simulink model "LQR_Control_Model"  (R2018b)
settings: Solver=ode1  StartTime=0.0  StopTime=15  FixedStep=0.001  MaxStep=0.001  RelTol=1e-3
values from neighbouring files (symbols this model uses):
  K = 0.2    [SingleNN_Delta.m]    (also in SingleNN_Hebb.m)
undefined symbols (not defined in the file or in its folder): sigbuilder_block
settings Model: Creator=Lenovo  LastModifiedBy=Richard
settings DataIOCC: LimitDataPoints=on  SaveFormat=Array
settings OptimizationCC: BlockReduction=off  BooleanDataType=off  LifeSpan=inf
settings DebuggingCC: SaveWithParameterizedLinksMsg=none  UnderspecifiedInitializationDetection=Classic  MergeDetectMultiDrivingBlocksExec=none  SignalResolutionControl=TryResolveAllWithWarning  SFUnexpectedBacktrackingDiag=warning  SFNoUnconditionalDefaultTransitionDiag=warning  SFExecutionAtInitializationDiag=none
settings HardwareCC: ProdBitPerPointer=32  ProdBitPerSizeT=32  ProdBitPerPtrDiffT=32  ProdLargestAtomicFloat=None  ProdIntDivRoundTo=Undefined  ProdEndianess=Unspecified  ProdWordSize=32  ProdHWDeviceType=32-bit Generic  TargetUnknown=on
settings ModelReferenceCC: PropagateSignalLabelsOutOfModel=off
settings SFSimCC: SimUseLocalCustomCode=off
settings RTWCC: RTWUseLocalCustomCode=off
settings CodeAppCC: StateflowObjectComments=on
settings GRTTargetCC: TargetLangStandard=C89/C90 (ANSI)  GeneratePreprocessorConditionals=Disable all
settings ConfigComp: CovMetricSettings=dw  CovHtmlReporting=on  CovSaveCumulativeToWorkspaceVar=on  CovSaveSingleToWorkspaceVar=on  CovExternalEMLEnable=off  CovSFcnEnable=off

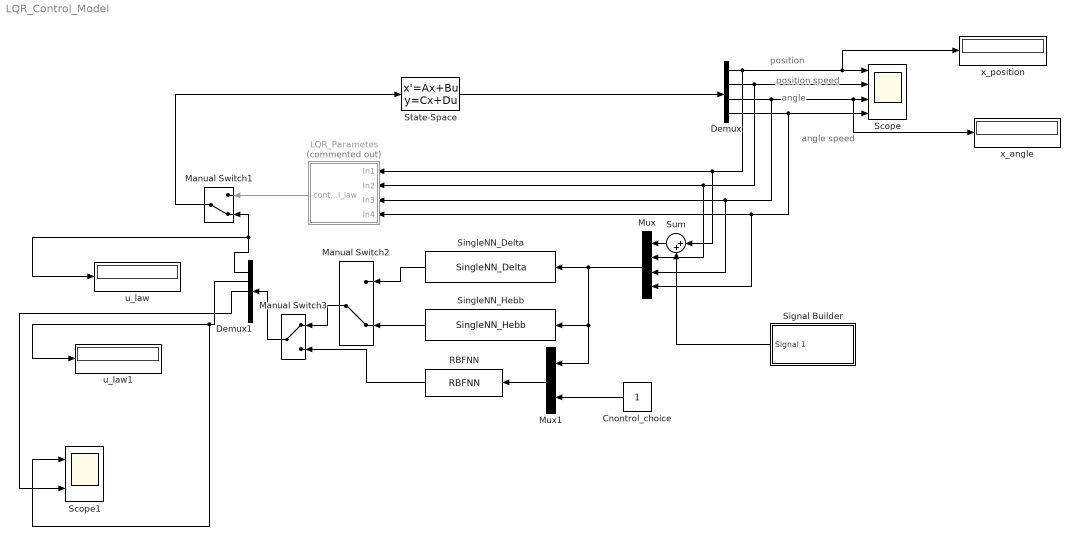
== system LQR_Control_Model ==
  note: angle speed
  note: angle
  note: position speed
  note: position
  Cnontrol_choice : Constant
  Demux : Demux
  Demux1 : Demux  Outputs=5
  LQR_Parametes : Subsystem  Commented=on
  Manual Switch1 : ManualSwitch  CurrentSetting=0
  Manual Switch2 : ManualSwitch  CurrentSetting=0
  Manual Switch3 : ManualSwitch
  Mux : Mux
  Mux1 : Mux  Inputs=2
  RBFNN : S-Function  FunctionName=RBFNN  SFunctionDeploymentMode=off  EnableBusSupport=off
  Scope : Scope  NumInputPorts=4
  Scope1 : Scope  NumInputPorts=2
  Signal Builder : Subsystem  Tag=STV Subsys  LoadFcn=sigbuilder_block('load',[437.6 199.2 550.4 400 ]);  StartFcn=sigbuilder_block('start');  StopFcn=sigbuilder_block('stop');  ClipboardFcn=sigbuilder_block('clipboard');  mask(Sigbuilder block){tuvar=[0:10]}
      mask help: Simulink:masks:SigbuilderBlock_MD
      mask init:
      | if ~strcmp(get_param(bdroot(gcbh),'SimulationStatus'),'stopped') tuvar = sigbuilder_block('maskInit'); end
      settings: CopyFcn=sigbuilder_block('copy');  DeleteFcn=sigbuilder_block('delete');  ModelCloseFcn=sigbuilder_block('modelClose');  PreSaveFcn=sigbuilder_block('preSave');  PauseFcn=sigbuilder_block('pause');  ContinueFcn=sigbuilder_block('continue');  NameChangeFcn=sigbuilder_block('namechange');  OpenFcn=sigbuilder_block('open',[437.6 199.2 550.4 400 ]);  CloseFcn=sigbuilder_block('close');
      mask Display: plot(0, 0, 100, 100,[2, 2, 32, 32, 2], [68, 8, 8, 68, 68],[32, 2], [38, 38], [32, 19, 2],[53, 60, 44], [32, 17, 17, 2],[16, 16, 31, 31]);txt = getActiveGroup(gcbh);text(2, 100, txt,'verticalAlignment', 'top');
  SingleNN_Delta : S-Function  FunctionName=SingleNN_Delta  SFunctionDeploymentMode=off  EnableBusSupport=off
  SingleNN_Hebb : S-Function  FunctionName=SingleNN_Hebb  SFunctionDeploymentMode=off  EnableBusSupport=off
  State-Space : StateSpace  A=[0 1 0 0;0 -0.1164 1.2373 0;0 0 0 1;0 -0.7164 67.9221 0]  B=[0;1.4554;0;8.9546]  C=[1 0 0 0;0 1 0 0;0 0 1 0;0 0 0 1]  D=[0;0;0;0]  InitialCondition=[1;1;1;1]
  Sum : Sum  Inputs=|++
  u_law : Display
  u_law1 : Display
  x_angle : Display
  x_position : Display
  wires:
  State-Space/1 -> Demux/1
  Demux/1 -> Sum/1, LQR_Parametes/1(In1), x_position/1, Scope/1
  Demux/2 -> LQR_Parametes/2(In2), Mux/2, Scope/2
  Demux/4 -> LQR_Parametes/4(In4), Mux/4, Scope/4
  LQR_Parametes/1(control_law) -> Manual Switch1/1
  Demux/3 -> LQR_Parametes/3(In3), Mux/3, x_angle/1, Scope/3
  Demux1/1 -> Manual Switch1/2, u_law/1
  Manual Switch1/1 -> State-Space/1
  SingleNN_Delta/1 -> Manual Switch2/1
  SingleNN_Hebb/1 -> Manual Switch2/2
  Mux/1 -> Mux1/1, SingleNN_Hebb/1, SingleNN_Delta/1
  Manual Switch3/1 -> Demux1/1
  Manual Switch2/1 -> Manual Switch3/1
  RBFNN/1 -> Manual Switch3/2
  Cnontrol_choice/1 -> Mux1/2
  Mux1/1 -> RBFNN/1
  Demux1/2 -> Scope1/1, u_law1/1
  Demux1/3 -> Scope1/2
  Sum/1 -> Mux/1
  Signal Builder/1(Signal 1) -> Sum/2

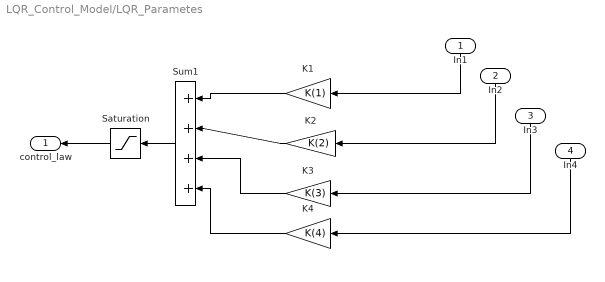
== system LQR_Control_Model/LQR_Parametes ==
  In1 : Inport
  In2 : Inport  Port=2
  In3 : Inport  Port=3
  In4 : Inport  Port=4
  K1 : Gain  Gain=K(1)
  K2 : Gain  Gain=K(2)
  K3 : Gain  Gain=K(3)
  K4 : Gain  Gain=K(4)
  Saturation : Saturate  UpperLimit=10  LowerLimit=-10
  Sum1 : Sum  Inputs=|++++
  control_law : Outport
  wires:
  In1/1 -> K1/1
  In3/1 -> K3/1
  In4/1 -> K4/1
  In2/1 -> K2/1
  K2/1 -> Sum1/2
  K1/1 -> Sum1/1
  K3/1 -> Sum1/3
  K4/1 -> Sum1/4
  Sum1/1 -> Saturation/1
  Saturation/1 -> control_law/1

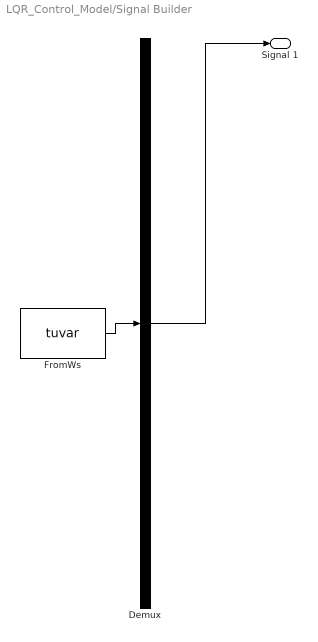
== system LQR_Control_Model/Signal Builder ==
  Demux : Demux  Tag=STV Demux  Outputs=1
  FromWs : FromWorkspace  Tag=STV FromWs  VariableName=tuvar  SampleTime=0
      SigBuilderData=|
      | common.afterFinalStr = 'Extrapolate'
      | common.sampleTime = 0
      | dataSet.timeRange = [0 10]
      | dataSet.name = 'Group 1'
      | sbobj.Groups.Name = 'Group 1'
      | sbobj.Groups.Signals.Name = 'Signal 1'
      | sbobj.Groups.Signals.XData = [0 4 4 10]
      | sbobj.Groups.Signals.YData = [0 0 1 1]
  Signal 1 : Outport  Tag=STV Outport
  wires:
  Demux/1 -> Signal 1/1
  FromWs/1 -> Demux/1
